simulink model "up1"  (R2018a)
settings: Solver=VariableStepAuto  StartTime=0.0  StopTime=100  RelTol=1e-3
undefined symbols (not defined in the file): m, n
settings Model: Creator=User  LastModifiedBy=User

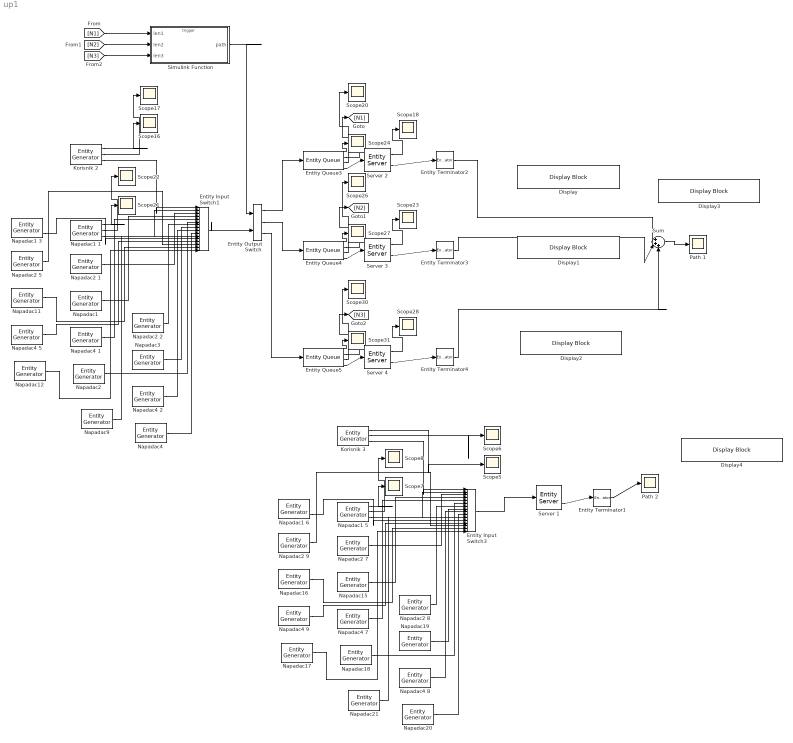
== system up1 ==
  Display : DisplayBlock  WebBlockId=49  LabelPosition=Hide
  Display1 : DisplayBlock  WebBlockId=50  LabelPosition=Hide
  Display2 : DisplayBlock  WebBlockId=51  LabelPosition=Hide
  Display3 : DisplayBlock  WebBlockId=57  LabelPosition=Hide
  Display4 : DisplayBlock  WebBlockId=62  LabelPosition=Hide
  Entity Input Switch1 : EntityInputSwitch  InputPortMessageModes=m,m,m,m,m,m,m,m,m,m,m,m,m,m,m,m  OutputPortMessageModes=m  NumberInputPorts=16
      settings: InputPortMap=u1,u2,u3,u4,u5,u6,u7,u8,u9,u10,u11,u12,u13,u14,u15,u16
  Entity Input Switch3 : EntityInputSwitch  InputPortMessageModes=m,m,m,m,m,m,m,m,m,m,m,m,m,m,m,m  OutputPortMessageModes=m  NumberInputPorts=16
      settings: InputPortMap=u1,u2,u3,u4,u5,u6,u7,u8,u9,u10,u11,u12,u13,u14,u15,u16
  Entity Output Switch : EntityOutputSwitch  InputPortMessageModes=m,m  OutputPortMessageModes=m,m,m  NumberOutputPorts=3  SwitchingCriterion=From control port  SwitchAttributeName=Attribute1
      settings: InputPortMap=u0,u1  OutputPortMap=o0,o1,o2
  Entity Queue3 : EntityQueue  InputPortMessageModes=m  OutputPortMessageModes=n,n,n,m  Capacity=500  NumberEntitiesDeparted=on  NumberEntitiesInBlock=on  AverageWait=on
      settings: OutputPortMap=o0,o1,o2,o5
  Entity Queue4 : EntityQueue  InputPortMessageModes=m  OutputPortMessageModes=n,n,n,m  Capacity=500  NumberEntitiesDeparted=on  NumberEntitiesInBlock=on  AverageWait=on
      settings: OutputPortMap=o0,o1,o2,o5
  Entity Queue5 : EntityQueue  InputPortMessageModes=m  OutputPortMessageModes=n,n,n,m  Capacity=500  NumberEntitiesDeparted=on  NumberEntitiesInBlock=on  AverageWait=on
      settings: OutputPortMap=o0,o1,o2,o5
  Entity Terminator{1..4} (4 alike) : EntityTerminator  InputPortMessageModes=m  NumberEntitiesArrived=on
      settings: OutputPortMap=o0
  Korisnik 2 : EntityGenerator  OutputPortMessageModes=n,n,m  TimeSource=MATLAB action  IntergenerationTimeAction=|  GenerateAction=|  AttributeName=vrijeme  AttributeInitialValue=0  NumberEntitiesDeparted=on  AverageIntergenerationTime=on  EntityType=Structured  EntityTypeName=vrijeme  DataInitialValue=1
      | persistent rngInit;
      | if isempty(rngInit)
      |     seed = 12345;
      |     rng(seed);
      |     rngInit = true;
      | end
      | 
      | % Pattern: Uniform distribution
      | % m: Minimum, M: Maximum
      | m = 0.1, M = 1;
      | dt = m + (M - m) * rand;
      | persistent rngInit;
      | if isempty(rngInit)
      |     seed = 12345;
      |     rng(seed);
      |     rngInit = true;
      | end
      | computeRouting();
      | % Pattern: Uniform distribution
      | % m: Minimum, M: Maximum
      | m = 0.1, M = 0.5;
      | entity.vrijeme = m + (M - m) * rand;
      settings: OutputPortMap=o0,o2,o3
  Korisnik 3 : EntityGenerator  OutputPortMessageModes=n,n,m  TimeSource=MATLAB action  IntergenerationTimeAction=|  GenerateAction=|  AttributeName=vrijeme  AttributeInitialValue=0  NumberEntitiesDeparted=on  AverageIntergenerationTime=on  EntityType=Structured  EntityTypeName=vrijeme  DataInitialValue=1
      | persistent rngInit;
      | if isempty(rngInit)
      |     seed = 12345;
      |     rng(seed);
      |     rngInit = true;
      | end
      | 
      | % Pattern: Uniform distribution
      | % m: Minimum, M: Maximum
      | m = 0.1, M = 1;
      | dt = m + (M - m) * rand;
      | persistent rngInit;
      | if isempty(rngInit)
      |     seed = 12345;
      |     rng(seed);
      |     rngInit = true;
      | end
      | computeRouting();
      | % Pattern: Uniform distribution
      | % m: Minimum, M: Maximum
      | m = 0.1, M = 0.5;
      | entity.vrijeme = m + (M - m) * rand;
      settings: OutputPortMap=o0,o2,o3
  Napadac1 : EntityGenerator  OutputPortMessageModes=m  TimeSource=MATLAB action  IntergenerationTimeAction=|  GenerateAction=|  AttributeName=vrijeme  AttributeInitialValue=0  EntityType=Structured  EntityTypeName=vrijeme  DataInitialValue=1
      | persistent rngInit;
      | if isempty(rngInit)
      |     seed = 12345;
      |     rng(seed);
      |     rngInit = true;
      | end
      | 
      | % Pattern: Uniform distribution
      | % m: Minimum, M: Maximum
      | m = 0.005, M = 0.02;
      | dt = m + (M - m) * rand;
      | computeRouting();
      | persistent rngInit;
      | if isempty(rngInit)
      |     seed = 12345;
      |     rng(seed);
      |     rngInit = true;
      | end
      | 
      | % Pattern: Uniform distribution
      | % m: Minimum, M: Maximum
      | m = 0.005, M = 0.02;
      | entity.vrijeme = m + (M - m) * rand;
  Napadac1 1 : EntityGenerator  OutputPortMessageModes=n,n,m  TimeSource=MATLAB action  IntergenerationTimeAction=|  GenerateAction=|  AttributeName=vrijeme  AttributeInitialValue=0  NumberEntitiesDeparted=on  AverageIntergenerationTime=on  EntityType=Structured  EntityTypeName=vrijeme  DataInitialValue=1
      | persistent rngInit;
      | if isempty(rngInit)
      |     seed = 12345;
      |     rng(seed);
      |     rngInit = true;
      | end
      | 
      | % Pattern: Uniform distribution
      | % m: Minimum, M: Maximum
      | m = 0.005, M = 0.02;
      | dt = m + (M - m) * rand;
      | persistent rngInit;
      | if isempty(rngInit)
      |     seed = 12345;
      |     rng(seed);
      |     rngInit = true;
      | end
      | computeRouting();
      | % Pattern: Uniform distribution
      | % m: Minimum, M: Maximum
      | m = 0.005, M = 0.02;
      | entity.vrijeme = m + (M - m) * rand;
      settings: OutputPortMap=o0,o2,o3
  Napadac1 3 : EntityGenerator  OutputPortMessageModes=n,n,m  TimeSource=MATLAB action  IntergenerationTimeAction=|  GenerateAction=|  AttributeName=vrijeme  AttributeInitialValue=0  NumberEntitiesDeparted=on  AverageIntergenerationTime=on  EntityType=Structured  EntityTypeName=vrijeme  DataInitialValue=1
      | persistent rngInit;
      | if isempty(rngInit)
      |     seed = 12345;
      |     rng(seed);
      |     rngInit = true;
      | end
      | 
      | % Pattern: Uniform distribution
      | % m: Minimum, M: Maximum
      | m = 0.005, M = 0.02;
      | dt = m + (M - m) * rand;
      | persistent rngInit;
      | if isempty(rngInit)
      |     seed = 12345;
      |     rng(seed);
      |     rngInit = true;
      | end
      | computeRouting();
      | % Pattern: Uniform distribution
      | % m: Minimum, M: Maximum
      | m = 0.005, M = 0.02;
      | entity.vrijeme = m + (M - m) * rand;
      settings: OutputPortMap=o0,o2,o3
  Napadac1 5 : EntityGenerator  OutputPortMessageModes=n,n,m  TimeSource=MATLAB action  IntergenerationTimeAction=|  GenerateAction=|  AttributeName=vrijeme  AttributeInitialValue=0  NumberEntitiesDeparted=on  AverageIntergenerationTime=on  EntityType=Structured  EntityTypeName=vrijeme  DataInitialValue=1
      | persistent rngInit;
      | if isempty(rngInit)
      |     seed = 12345;
      |     rng(seed);
      |     rngInit = true;
      | end
      | 
      | % Pattern: Uniform distribution
      | % m: Minimum, M: Maximum
      | m = 0.005, M = 0.02;
      | dt = m + (M - m) * rand;
      | persistent rngInit;
      | if isempty(rngInit)
      |     seed = 12345;
      |     rng(seed);
      |     rngInit = true;
      | end
      | computeRouting();
      | % Pattern: Uniform distribution
      | % m: Minimum, M: Maximum
      | m = 0.005, M = 0.02;
      | entity.vrijeme = m + (M - m) * rand;
      settings: OutputPortMap=o0,o2,o3
  Napadac1 6 : EntityGenerator  OutputPortMessageModes=n,n,m  TimeSource=MATLAB action  IntergenerationTimeAction=|  GenerateAction=|  AttributeName=vrijeme  AttributeInitialValue=0  NumberEntitiesDeparted=on  AverageIntergenerationTime=on  EntityType=Structured  EntityTypeName=vrijeme  DataInitialValue=1
      | persistent rngInit;
      | if isempty(rngInit)
      |     seed = 12345;
      |     rng(seed);
      |     rngInit = true;
      | end
      | 
      | % Pattern: Uniform distribution
      | % m: Minimum, M: Maximum
      | m = 0.005, M = 0.02;
      | dt = m + (M - m) * rand;
      | persistent rngInit;
      | if isempty(rngInit)
      |     seed = 12345;
      |     rng(seed);
      |     rngInit = true;
      | end
      | computeRouting();
      | % Pattern: Uniform distribution
      | % m: Minimum, M: Maximum
      | m = 0.005, M = 0.02;
      | entity.vrijeme = m + (M - m) * rand;
      settings: OutputPortMap=o0,o2,o3
  Napadac11 : EntityGenerator  OutputPortMessageModes=m  TimeSource=MATLAB action  IntergenerationTimeAction=|  GenerateAction=|  AttributeName=vrijeme  AttributeInitialValue=0  EntityType=Structured  EntityTypeName=vrijeme  DataInitialValue=1
      | persistent rngInit;
      | if isempty(rngInit)
      |     seed = 12345;
      |     rng(seed);
      |     rngInit = true;
      | end
      | 
      | % Pattern: Uniform distribution
      | % m: Minimum, M: Maximum
      | m = 0.005, M = 0.02;
      | dt = m + (M - m) * rand;
      | computeRouting();
      | persistent rngInit;
      | if isempty(rngInit)
      |     seed = 12345;
      |     rng(seed);
      |     rngInit = true;
      | end
      | 
      | % Pattern: Uniform distribution
      | % m: Minimum, M: Maximum
      | m = 0.005, M = 0.02;
      | entity.vrijeme = m + (M - m) * rand;
  Napadac12 : EntityGenerator  OutputPortMessageModes=m  TimeSource=MATLAB action  IntergenerationTimeAction=|  GenerateAction=|  AttributeName=vrijeme  AttributeInitialValue=0  EntityType=Structured  EntityTypeName=vrijeme  DataInitialValue=1
      | persistent rngInit;
      | if isempty(rngInit)
      |     seed = 12345;
      |     rng(seed);
      |     rngInit = true;
      | end
      | 
      | % Pattern: Uniform distribution
      | % m: Minimum, M: Maximum
      | m = 0.005, M = 0.02;
      | dt = m + (M - m) * rand;
      | computeRouting();
      | persistent rngInit;
      | if isempty(rngInit)
      |     seed = 12345;
      |     rng(seed);
      |     rngInit = true;
      | end
      | 
      | % Pattern: Uniform distribution
      | % m: Minimum, M: Maximum
      | m = 0.005, M = 0.02;
      | entity.vrijeme = m + (M - m) * rand;
  Napadac15 : EntityGenerator  OutputPortMessageModes=m  TimeSource=MATLAB action  IntergenerationTimeAction=|  GenerateAction=|  AttributeName=vrijeme  AttributeInitialValue=0  EntityType=Structured  EntityTypeName=vrijeme  DataInitialValue=1
      | persistent rngInit;
      | if isempty(rngInit)
      |     seed = 12345;
      |     rng(seed);
      |     rngInit = true;
      | end
      | 
      | % Pattern: Uniform distribution
      | % m: Minimum, M: Maximum
      | m = 0.005, M = 0.02;
      | dt = m + (M - m) * rand;
      | computeRouting();
      | persistent rngInit;
      | if isempty(rngInit)
      |     seed = 12345;
      |     rng(seed);
      |     rngInit = true;
      | end
      | 
      | % Pattern: Uniform distribution
      | % m: Minimum, M: Maximum
      | m = 0.005, M = 0.02;
      | entity.vrijeme = m + (M - m) * rand;
  Napadac16 : EntityGenerator  OutputPortMessageModes=m  TimeSource=MATLAB action  IntergenerationTimeAction=|  GenerateAction=|  AttributeName=vrijeme  AttributeInitialValue=0  EntityType=Structured  EntityTypeName=vrijeme  DataInitialValue=1
      | persistent rngInit;
      | if isempty(rngInit)
      |     seed = 12345;
      |     rng(seed);
      |     rngInit = true;
      | end
      | 
      | % Pattern: Uniform distribution
      | % m: Minimum, M: Maximum
      | m = 0.005, M = 0.02;
      | dt = m + (M - m) * rand;
      | computeRouting();
      | persistent rngInit;
      | if isempty(rngInit)
      |     seed = 12345;
      |     rng(seed);
      |     rngInit = true;
      | end
      | 
      | % Pattern: Uniform distribution
      | % m: Minimum, M: Maximum
      | m = 0.005, M = 0.02;
      | entity.vrijeme = m + (M - m) * rand;
  Napadac17 : EntityGenerator  OutputPortMessageModes=m  TimeSource=MATLAB action  IntergenerationTimeAction=|  GenerateAction=|  AttributeName=vrijeme  AttributeInitialValue=0  EntityType=Structured  EntityTypeName=vrijeme  DataInitialValue=1
      | persistent rngInit;
      | if isempty(rngInit)
      |     seed = 12345;
      |     rng(seed);
      |     rngInit = true;
      | end
      | 
      | % Pattern: Uniform distribution
      | % m: Minimum, M: Maximum
      | m = 0.005, M = 0.02;
      | dt = m + (M - m) * rand;
      | computeRouting();
      | persistent rngInit;
      | if isempty(rngInit)
      |     seed = 12345;
      |     rng(seed);
      |     rngInit = true;
      | end
      | 
      | % Pattern: Uniform distribution
      | % m: Minimum, M: Maximum
      | m = 0.005, M = 0.02;
      | entity.vrijeme = m + (M - m) * rand;
  Napadac18 : EntityGenerator  OutputPortMessageModes=m  TimeSource=MATLAB action  IntergenerationTimeAction=|  GenerateAction=|  AttributeName=vrijeme  AttributeInitialValue=0  EntityType=Structured  EntityTypeName=vrijeme  DataInitialValue=1
      | persistent rngInit;
      | if isempty(rngInit)
      |     seed = 12345;
      |     rng(seed);
      |     rngInit = true;
      | end
      | 
      | % Pattern: Uniform distribution
      | % m: Minimum, M: Maximum
      | m = 0.005, M = 0.02;
      | dt = m + (M - m) * rand;
      | computeRouting();
      | persistent rngInit;
      | if isempty(rngInit)
      |     seed = 12345;
      |     rng(seed);
      |     rngInit = true;
      | end
      | 
      | % Pattern: Uniform distribution
      | % m: Minimum, M: Maximum
      | m = 0.005, M = 0.02;
      | entity.vrijeme = m + (M - m) * rand;
  Napadac19 : EntityGenerator  OutputPortMessageModes=m  TimeSource=MATLAB action  IntergenerationTimeAction=|  GenerateAction=|  AttributeName=vrijeme  AttributeInitialValue=0  EntityType=Structured  EntityTypeName=vrijeme  DataInitialValue=1
      | persistent rngInit;
      | if isempty(rngInit)
      |     seed = 12345;
      |     rng(seed);
      |     rngInit = true;
      | end
      | 
      | % Pattern: Uniform distribution
      | % m: Minimum, M: Maximum
      | m = 0.005, M = 0.02;
      | dt = m + (M - m) * rand;
      | computeRouting();
      | persistent rngInit;
      | if isempty(rngInit)
      |     seed = 12345;
      |     rng(seed);
      |     rngInit = true;
      | end
      | 
      | % Pattern: Uniform distribution
      | % m: Minimum, M: Maximum
      | m = 0.005, M = 0.02;
      | entity.vrijeme = m + (M - m) * rand;
  Napadac2 : EntityGenerator  OutputPortMessageModes=m  TimeSource=MATLAB action  IntergenerationTimeAction=|  GenerateAction=|  AttributeName=vrijeme  AttributeInitialValue=0  EntityType=Structured  EntityTypeName=vrijeme  DataInitialValue=1
      | persistent rngInit;
      | if isempty(rngInit)
      |     seed = 12345;
      |     rng(seed);
      |     rngInit = true;
      | end
      | 
      | % Pattern: Uniform distribution
      | % m: Minimum, M: Maximum
      | m = 0.005, M = 0.02;
      | dt = m + (M - m) * rand;
      | computeRouting();
      | persistent rngInit;
      | if isempty(rngInit)
      |     seed = 12345;
      |     rng(seed);
      |     rngInit = true;
      | end
      | 
      | % Pattern: Uniform distribution
      | % m: Minimum, M: Maximum
      | m = 0.005, M = 0.02;
      | entity.vrijeme = m + (M - m) * rand;
  Napadac2 1 : EntityGenerator  OutputPortMessageModes=m  TimeSource=MATLAB action  IntergenerationTimeAction=|  GenerateAction=|  AttributeName=vrijeme  AttributeInitialValue=0  EntityType=Structured  EntityTypeName=vrijeme  DataInitialValue=1
      | persistent rngInit;
      | if isempty(rngInit)
      |     seed = 12345;
      |     rng(seed);
      |     rngInit = true;
      | end
      | 
      | % Pattern: Uniform distribution
      | % m: Minimum, M: Maximum
      | m = 0.005, M = 0.02;
      | dt = m + (M - m) * rand;
      | computeRouting();
      | persistent rngInit;
      | if isempty(rngInit)
      |     seed = 12345;
      |     rng(seed);
      |     rngInit = true;
      | end
      | 
      | % Pattern: Uniform distribution
      | % m: Minimum, M: Maximum
      | m = 0.005, M = 0.02;
      | entity.vrijeme = m + (M - m) * rand;
  Napadac2 2 : EntityGenerator  OutputPortMessageModes=m  TimeSource=MATLAB action  IntergenerationTimeAction=|  GenerateAction=|  AttributeName=vrijeme  AttributeInitialValue=0  EntityType=Structured  EntityTypeName=vrijeme  DataInitialValue=1
      | persistent rngInit;
      | if isempty(rngInit)
      |     seed = 12345;
      |     rng(seed);
      |     rngInit = true;
      | end
      | 
      | % Pattern: Uniform distribution
      | % m: Minimum, M: Maximum
      | m = 0.005, M = 0.02;
      | dt = m + (M - m) * rand;
      | computeRouting();
      | persistent rngInit;
      | if isempty(rngInit)
      |     seed = 12345;
      |     rng(seed);
      |     rngInit = true;
      | end
      | 
      | % Pattern: Uniform distribution
      | % m: Minimum, M: Maximum
      | m = 0.005, M = 0.02;
      | entity.vrijeme = m + (M - m) * rand;
  Napadac2 5 : EntityGenerator  OutputPortMessageModes=m  TimeSource=MATLAB action  IntergenerationTimeAction=|  GenerateAction=|  AttributeName=vrijeme  AttributeInitialValue=0  EntityType=Structured  EntityTypeName=vrijeme  DataInitialValue=1
      | persistent rngInit;
      | if isempty(rngInit)
      |     seed = 12345;
      |     rng(seed);
      |     rngInit = true;
      | end
      | 
      | % Pattern: Uniform distribution
      | % m: Minimum, M: Maximum
      | m = 0.005, M = 0.02;
      | dt = m + (M - m) * rand;
      | computeRouting();
      | persistent rngInit;
      | if isempty(rngInit)
      |     seed = 12345;
      |     rng(seed);
      |     rngInit = true;
      | end
      | 
      | % Pattern: Uniform distribution
      | % m: Minimum, M: Maximum
      | m = 0.005, M = 0.02;
      | entity.vrijeme = m + (M - m) * rand;
  Napadac2 7 : EntityGenerator  OutputPortMessageModes=m  TimeSource=MATLAB action  IntergenerationTimeAction=|  GenerateAction=|  AttributeName=vrijeme  AttributeInitialValue=0  EntityType=Structured  EntityTypeName=vrijeme  DataInitialValue=1
      | persistent rngInit;
      | if isempty(rngInit)
      |     seed = 12345;
      |     rng(seed);
      |     rngInit = true;
      | end
      | 
      | % Pattern: Uniform distribution
      | % m: Minimum, M: Maximum
      | m = 0.005, M = 0.02;
      | dt = m + (M - m) * rand;
      | computeRouting();
      | persistent rngInit;
      | if isempty(rngInit)
      |     seed = 12345;
      |     rng(seed);
      |     rngInit = true;
      | end
      | 
      | % Pattern: Uniform distribution
      | % m: Minimum, M: Maximum
      | m = 0.005, M = 0.02;
      | entity.vrijeme = m + (M - m) * rand;
  Napadac2 8 : EntityGenerator  OutputPortMessageModes=m  TimeSource=MATLAB action  IntergenerationTimeAction=|  GenerateAction=|  AttributeName=vrijeme  AttributeInitialValue=0  EntityType=Structured  EntityTypeName=vrijeme  DataInitialValue=1
      | persistent rngInit;
      | if isempty(rngInit)
      |     seed = 12345;
      |     rng(seed);
      |     rngInit = true;
      | end
      | 
      | % Pattern: Uniform distribution
      | % m: Minimum, M: Maximum
      | m = 0.005, M = 0.02;
      | dt = m + (M - m) * rand;
      | computeRouting();
      | persistent rngInit;
      | if isempty(rngInit)
      |     seed = 12345;
      |     rng(seed);
      |     rngInit = true;
      | end
      | 
      | % Pattern: Uniform distribution
      | % m: Minimum, M: Maximum
      | m = 0.005, M = 0.02;
      | entity.vrijeme = m + (M - m) * rand;
  Napadac2 9 : EntityGenerator  OutputPortMessageModes=m  TimeSource=MATLAB action  IntergenerationTimeAction=|  GenerateAction=|  AttributeName=vrijeme  AttributeInitialValue=0  EntityType=Structured  EntityTypeName=vrijeme  DataInitialValue=1
      | persistent rngInit;
      | if isempty(rngInit)
      |     seed = 12345;
      |     rng(seed);
      |     rngInit = true;
      | end
      | 
      | % Pattern: Uniform distribution
      | % m: Minimum, M: Maximum
      | m = 0.005, M = 0.02;
      | dt = m + (M - m) * rand;
      | computeRouting();
      | persistent rngInit;
      | if isempty(rngInit)
      |     seed = 12345;
      |     rng(seed);
      |     rngInit = true;
      | end
      | 
      | % Pattern: Uniform distribution
      | % m: Minimum, M: Maximum
      | m = 0.005, M = 0.02;
      | entity.vrijeme = m + (M - m) * rand;
  Napadac20 : EntityGenerator  OutputPortMessageModes=m  TimeSource=MATLAB action  IntergenerationTimeAction=|  GenerateAction=|  AttributeName=vrijeme  AttributeInitialValue=0  EntityType=Structured  EntityTypeName=vrijeme  DataInitialValue=1
      | persistent rngInit;
      | if isempty(rngInit)
      |     seed = 12345;
      |     rng(seed);
      |     rngInit = true;
      | end
      | 
      | % Pattern: Uniform distribution
      | % m: Minimum, M: Maximum
      | m = 0.005, M = 0.02;
      | dt = m + (M - m) * rand;
      | computeRouting();
      | persistent rngInit;
      | if isempty(rngInit)
      |     seed = 12345;
      |     rng(seed);
      |     rngInit = true;
      | end
      | 
      | % Pattern: Uniform distribution
      | % m: Minimum, M: Maximum
      | m = 0.005, M = 0.02;
      | entity.vrijeme = m + (M - m) * rand;
  Napadac21 : EntityGenerator  OutputPortMessageModes=m  TimeSource=MATLAB action  IntergenerationTimeAction=|  GenerateAction=|  AttributeName=vrijeme  AttributeInitialValue=0  EntityType=Structured  EntityTypeName=vrijeme  DataInitialValue=1
      | persistent rngInit;
      | if isempty(rngInit)
      |     seed = 12345;
      |     rng(seed);
      |     rngInit = true;
      | end
      | 
      | % Pattern: Uniform distribution
      | % m: Minimum, M: Maximum
      | m = 0.005, M = 0.02;
      | dt = m + (M - m) * rand;
      | computeRouting();
      | persistent rngInit;
      | if isempty(rngInit)
      |     seed = 12345;
      |     rng(seed);
      |     rngInit = true;
      | end
      | 
      | % Pattern: Uniform distribution
      | % m: Minimum, M: Maximum
      | m = 0.005, M = 0.02;
      | entity.vrijeme = m + (M - m) * rand;
  Napadac3 : EntityGenerator  OutputPortMessageModes=m  TimeSource=MATLAB action  IntergenerationTimeAction=|  GenerateAction=|  AttributeName=vrijeme  AttributeInitialValue=0  EntityType=Structured  EntityTypeName=vrijeme  DataInitialValue=1
      | persistent rngInit;
      | if isempty(rngInit)
      |     seed = 12345;
      |     rng(seed);
      |     rngInit = true;
      | end
      | 
      | % Pattern: Uniform distribution
      | % m: Minimum, M: Maximum
      | m = 0.005, M = 0.02;
      | dt = m + (M - m) * rand;
      | computeRouting();
      | persistent rngInit;
      | if isempty(rngInit)
      |     seed = 12345;
      |     rng(seed);
      |     rngInit = true;
      | end
      | 
      | % Pattern: Uniform distribution
      | % m: Minimum, M: Maximum
      | m = 0.005, M = 0.02;
      | entity.vrijeme = m + (M - m) * rand;
  Napadac4 : EntityGenerator  OutputPortMessageModes=m  TimeSource=MATLAB action  IntergenerationTimeAction=|  GenerateAction=|  AttributeName=vrijeme  AttributeInitialValue=0  EntityType=Structured  EntityTypeName=vrijeme  DataInitialValue=1
      | persistent rngInit;
      | if isempty(rngInit)
      |     seed = 12345;
      |     rng(seed);
      |     rngInit = true;
      | end
      | 
      | % Pattern: Uniform distribution
      | % m: Minimum, M: Maximum
      | m = 0.005, M = 0.02;
      | dt = m + (M - m) * rand;
      | computeRouting();
      | persistent rngInit;
      | if isempty(rngInit)
      |     seed = 12345;
      |     rng(seed);
      |     rngInit = true;
      | end
      | 
      | % Pattern: Uniform distribution
      | % m: Minimum, M: Maximum
      | m = 0.005, M = 0.02;
      | entity.vrijeme = m + (M - m) * rand;
  Napadac4 1 : EntityGenerator  OutputPortMessageModes=m  TimeSource=MATLAB action  IntergenerationTimeAction=|  GenerateAction=|  AttributeName=vrijeme  AttributeInitialValue=0  EntityType=Structured  EntityTypeName=vrijeme  DataInitialValue=1
      | persistent rngInit;
      | if isempty(rngInit)
      |     seed = 12345;
      |     rng(seed);
      |     rngInit = true;
      | end
      | 
      | % Pattern: Uniform distribution
      | % m: Minimum, M: Maximum
      | m = 0.005, M = 0.02;
      | dt = m + (M - m) * rand;
      | computeRouting();
      | persistent rngInit;
      | if isempty(rngInit)
      |     seed = 12345;
      |     rng(seed);
      |     rngInit = true;
      | end
      | 
      | % Pattern: Uniform distribution
      | % m: Minimum, M: Maximum
      | m = 0.005, M = 0.02;
      | entity.vrijeme = m + (M - m) * rand;
  Napadac4 2 : EntityGenerator  OutputPortMessageModes=m  TimeSource=MATLAB action  IntergenerationTimeAction=|  GenerateAction=|  AttributeName=vrijeme  AttributeInitialValue=0  EntityType=Structured  EntityTypeName=vrijeme  DataInitialValue=1
      | persistent rngInit;
      | if isempty(rngInit)
      |     seed = 12345;
      |     rng(seed);
      |     rngInit = true;
      | end
      | 
      | % Pattern: Uniform distribution
      | % m: Minimum, M: Maximum
      | m = 0.005, M = 0.02;
      | dt = m + (M - m) * rand;
      | computeRouting();
      | persistent rngInit;
      | if isempty(rngInit)
      |     seed = 12345;
      |     rng(seed);
      |     rngInit = true;
      | end
      | 
      | % Pattern: Uniform distribution
      | % m: Minimum, M: Maximum
      | m = 0.005, M = 0.02;
      | entity.vrijeme = m + (M - m) * rand;
  Napadac4 5 : EntityGenerator  OutputPortMessageModes=m  TimeSource=MATLAB action  IntergenerationTimeAction=|  GenerateAction=|  AttributeName=vrijeme  AttributeInitialValue=0  EntityType=Structured  EntityTypeName=vrijeme  DataInitialValue=1
      | persistent rngInit;
      | if isempty(rngInit)
      |     seed = 12345;
      |     rng(seed);
      |     rngInit = true;
      | end
      | 
      | % Pattern: Uniform distribution
      | % m: Minimum, M: Maximum
      | m = 0.005, M = 0.02;
      | dt = m + (M - m) * rand;
      | computeRouting();
      | persistent rngInit;
      | if isempty(rngInit)
      |     seed = 12345;
      |     rng(seed);
      |     rngInit = true;
      | end
      | 
      | % Pattern: Uniform distribution
      | % m: Minimum, M: Maximum
      | m = 0.005, M = 0.02;
      | entity.vrijeme = m + (M - m) * rand;
  Napadac4 7 : EntityGenerator  OutputPortMessageModes=m  TimeSource=MATLAB action  IntergenerationTimeAction=|  GenerateAction=|  AttributeName=vrijeme  AttributeInitialValue=0  EntityType=Structured  EntityTypeName=vrijeme  DataInitialValue=1
      | persistent rngInit;
      | if isempty(rngInit)
      |     seed = 12345;
      |     rng(seed);
      |     rngInit = true;
      | end
      | 
      | % Pattern: Uniform distribution
      | % m: Minimum, M: Maximum
      | m = 0.005, M = 0.02;
      | dt = m + (M - m) * rand;
      | computeRouting();
      | persistent rngInit;
      | if isempty(rngInit)
      |     seed = 12345;
      |     rng(seed);
      |     rngInit = true;
      | end
      | 
      | % Pattern: Uniform distribution
      | % m: Minimum, M: Maximum
      | m = 0.005, M = 0.02;
      | entity.vrijeme = m + (M - m) * rand;
  Napadac4 8 : EntityGenerator  OutputPortMessageModes=m  TimeSource=MATLAB action  IntergenerationTimeAction=|  GenerateAction=|  AttributeName=vrijeme  AttributeInitialValue=0  EntityType=Structured  EntityTypeName=vrijeme  DataInitialValue=1
      | persistent rngInit;
      | if isempty(rngInit)
      |     seed = 12345;
      |     rng(seed);
      |     rngInit = true;
      | end
      | 
      | % Pattern: Uniform distribution
      | % m: Minimum, M: Maximum
      | m = 0.005, M = 0.02;
      | dt = m + (M - m) * rand;
      | computeRouting();
      | persistent rngInit;
      | if isempty(rngInit)
      |     seed = 12345;
      |     rng(seed);
      |     rngInit = true;
      | end
      | 
      | % Pattern: Uniform distribution
      | % m: Minimum, M: Maximum
      | m = 0.005, M = 0.02;
      | entity.vrijeme = m + (M - m) * rand;
  Napadac4 9 : EntityGenerator  OutputPortMessageModes=m  TimeSource=MATLAB action  IntergenerationTimeAction=|  GenerateAction=|  AttributeName=vrijeme  AttributeInitialValue=0  EntityType=Structured  EntityTypeName=vrijeme  DataInitialValue=1
      | persistent rngInit;
      | if isempty(rngInit)
      |     seed = 12345;
      |     rng(seed);
      |     rngInit = true;
      | end
      | 
      | % Pattern: Uniform distribution
      | % m: Minimum, M: Maximum
      | m = 0.005, M = 0.02;
      | dt = m + (M - m) * rand;
      | computeRouting();
      | persistent rngInit;
      | if isempty(rngInit)
      |     seed = 12345;
      |     rng(seed);
      |     rngInit = true;
      | end
      | 
      | % Pattern: Uniform distribution
      | % m: Minimum, M: Maximum
      | m = 0.005, M = 0.02;
      | entity.vrijeme = m + (M - m) * rand;
  Napadac9 : EntityGenerator  OutputPortMessageModes=m  TimeSource=MATLAB action  IntergenerationTimeAction=|  GenerateAction=|  AttributeName=vrijeme  AttributeInitialValue=0  EntityType=Structured  EntityTypeName=vrijeme  DataInitialValue=1
      | persistent rngInit;
      | if isempty(rngInit)
      |     seed = 12345;
      |     rng(seed);
      |     rngInit = true;
      | end
      | 
      | % Pattern: Uniform distribution
      | % m: Minimum, M: Maximum
      | m = 0.005, M = 0.02;
      | dt = m + (M - m) * rand;
      | computeRouting();
      | persistent rngInit;
      | if isempty(rngInit)
      |     seed = 12345;
      |     rng(seed);
      |     rngInit = true;
      | end
      | 
      | % Pattern: Uniform distribution
      | % m: Minimum, M: Maximum
      | m = 0.005, M = 0.02;
      | entity.vrijeme = m + (M - m) * rand;
  Path 1 : Scope
  Path 2 : Scope
  Scope{5..8,16..18,20..24,26..28,30..31} (17 alike) : Scope
  Server 1 : EntityServer  InputPortMessageModes=m  OutputPortMessageModes=n,m  Capacity=inf  ServiceTimeSource=Attribute  ServiceTimeAttributeName=vrijeme  Utilization=on
      settings: OutputPortMap=o5,o9
  Server 2 : EntityServer  InputPortMessageModes=m  OutputPortMessageModes=n,m  Capacity=4  ServiceTimeSource=Attribute  ServiceTimeAttributeName=vrijeme  Utilization=on
      settings: OutputPortMap=o5,o9
  Server 3 : EntityServer  InputPortMessageModes=m  OutputPortMessageModes=n,m  Capacity=4  ServiceTimeSource=Attribute  ServiceTimeAttributeName=vrijeme  Utilization=on
      settings: OutputPortMap=o5,o9
  Server 4 : EntityServer  InputPortMessageModes=m  OutputPortMessageModes=n,m  Capacity=4  ServiceTimeSource=Attribute  ServiceTimeAttributeName=vrijeme  Utilization=on
      settings: OutputPortMap=o5,o9
  Simulink Function : Subsystem  TreatAsAtomicUnit=on
  Sum : Sum  Inputs=|+++
  wires:
  Server 2/1 -> Scope18/1
  Simulink Function/1(path) -> Entity Output Switch/1
  [N2] -> Simulink Function/2(len2)
  Entity Queue3/2 -> [N1]
  Entity Queue5/1 -> Scope31/1
  Napadac1 1/3 -> Entity Input Switch1/2
  [N1] -> Simulink Function/1(len1)
  Napadac2/1 -> Entity Input Switch1/6
  Entity Output Switch/2 -> Entity Queue4/1
  Server 4/2 -> Entity Terminator4/1
  Entity Queue5/4 -> Server 4/1
  Entity Queue5/3 -> Scope30/1
  Entity Queue3/3 -> Scope20/1
  Entity Output Switch/1 -> Entity Queue3/1
  Entity Queue4/3 -> Scope26/1
  Server 4/1 -> Scope28/1
  Entity Queue5/2 -> [N3]
  Server 3/2 -> Entity Terminator3/1
  Entity Output Switch/3 -> Entity Queue5/1
  Napadac1 1/1 -> Scope21/1
  Korisnik 2/2 -> Scope17/1
  [N3] -> Simulink Function/3(len3)
  Entity Queue4/2 -> [N2]
  Entity Input Switch1/1 -> Entity Output Switch/2
  Server 3/1 -> Scope23/1
  Korisnik 2/1 -> Scope16/1
  Entity Queue3/4 -> Server 2/1
  Entity Queue4/1 -> Scope27/1
  Napadac4 1/1 -> Entity Input Switch1/5
  Napadac1/1 -> Entity Input Switch1/4
  Server 2/2 -> Entity Terminator2/1
  Korisnik 2/3 -> Entity Input Switch1/1
  Entity Queue4/4 -> Server 3/1
  Napadac1 1/2 -> Scope22/1
  Entity Queue3/1 -> Scope24/1
  Napadac2 1/1 -> Entity Input Switch1/3
  Napadac2 2/1 -> Entity Input Switch1/7
  Napadac3/1 -> Entity Input Switch1/8
  Napadac4 2/1 -> Entity Input Switch1/9
  Napadac4/1 -> Entity Input Switch1/10
  Entity Terminator4/1 -> Sum/3
  Entity Terminator3/1 -> Sum/2
  Entity Terminator2/1 -> Sum/1
  Sum/1 -> Path 1/1
  Server 1/2 -> Entity Terminator1/1
  Entity Terminator1/1 -> Path 2/1
  Entity Input Switch3/1 -> Server 1/1
  Napadac9/1 -> Entity Input Switch1/11
  Napadac1 3/3 -> Entity Input Switch1/12
  Napadac2 5/1 -> Entity Input Switch1/14
  Napadac11/1 -> Entity Input Switch1/15
  Napadac4 5/1 -> Entity Input Switch1/13
  Napadac12/1 -> Entity Input Switch1/16
  Napadac2 9/1 -> Entity Input Switch3/14
  Napadac4 9/1 -> Entity Input Switch3/13
  Napadac17/1 -> Entity Input Switch3/16
  Korisnik 3/1 -> Scope5/1
  Napadac18/1 -> Entity Input Switch3/6
  Napadac20/1 -> Entity Input Switch3/10
  Korisnik 3/3 -> Entity Input Switch3/1
  Napadac2 7/1 -> Entity Input Switch3/3
  Napadac19/1 -> Entity Input Switch3/8
  Napadac2 8/1 -> Entity Input Switch3/7
  Napadac1 5/3 -> Entity Input Switch3/2
  Napadac16/1 -> Entity Input Switch3/15
  Napadac15/1 -> Entity Input Switch3/4
  Napadac4 7/1 -> Entity Input Switch3/5
  Napadac21/1 -> Entity Input Switch3/11
  Napadac4 8/1 -> Entity Input Switch3/9
  Napadac1 5/1 -> Scope7/1
  Napadac1 5/2 -> Scope8/1
  Korisnik 3/2 -> Scope6/1
  Napadac1 6/3 -> Entity Input Switch3/12

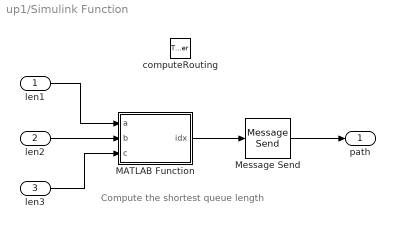
== system up1/Simulink Function ==
  note: Compute the shortest queue length
  len1 : Inport
  len2 : Inport  Port=2
  len3 : Inport  Port=3
  computeRouting : TriggerPort  TriggerType=function-call  IsSimulinkFunction=on  FunctionName=computeRouting  VariantControl=Variant
  MATLAB Function : MATLAB Function  TreatAsAtomicUnit=on
  Message Send : MessageSend  OutputPortMessageModes=m
      settings: InputPortMap=u1
  path : Outport
  wires:
  len1/1 -> MATLAB Function/1(a)
  len2/1 -> MATLAB Function/2(b)
  len3/1 -> MATLAB Function/3(c)
  MATLAB Function/1(idx) -> Message Send/1
  Message Send/1 -> path/1

== matlab function up1/Simulink Function/MATLAB Function ==
  data: a input; idx output; b input; c input
function idx = fcn(a,b,c)

[~, idx] = min([a,b,c]);
